simulink library "lib_plant"  (R2026a)
settings: Solver=VariableStepAuto
undefined symbols (not defined in the file or in its folder): zs0, zsdot0, zu0, zudot0
settings Model: Creator=alessandro-nardin  LastModifiedBy=alessandro-nardin

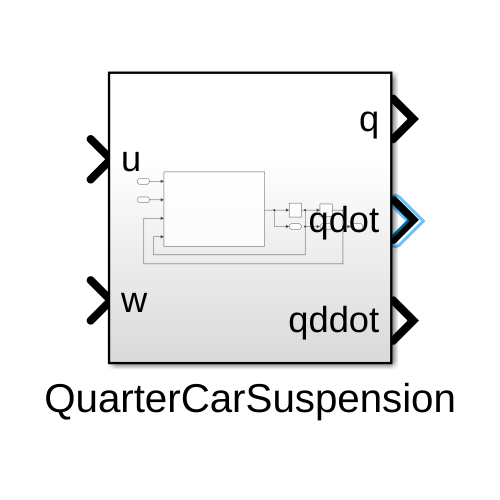
[thumbnail: Simulink's stored preview of the top-level diagram]
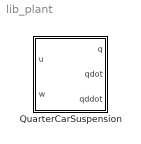
== system lib_plant ==
  QuarterCarSuspension : Subsystem

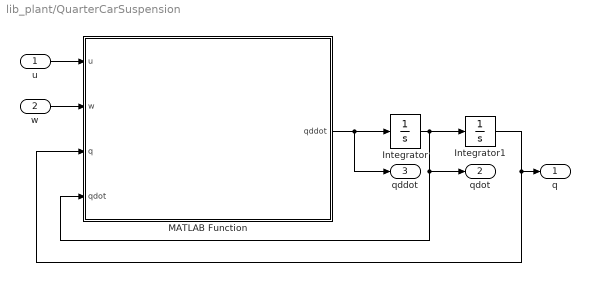
== system lib_plant/QuarterCarSuspension ==
  u : Inport
  w : Inport  Port=2
  Integrator : Integrator  InitialCondition=[ zsdot0; zudot0]
  Integrator1 : Integrator  InitialCondition=[ zs0; zu0 ]
  MATLAB Function : MATLAB Function  TreatAsAtomicUnit=on
  q : Outport
  qdot : Outport  Port=2
  qddot : Outport  Port=3
  wires:
  w/1 -> MATLAB Function/2(w)
  u/1 -> MATLAB Function/1(u)
  Integrator/1 -> qdot/1, MATLAB Function/4(qdot), Integrator1/1
  MATLAB Function/1(qddot) -> qddot/1, Integrator/1
  Integrator1/1 -> MATLAB Function/3(q), q/1

== matlab function lib_plant/QuarterCarSuspension/MATLAB Function ==
  data: u input size=[2 1]; w input size=[2 1]; q input size=[2 1]; qdot input size=[2 1]; qddot output size=[2 1]; plant_param parameter
function qddot = quarter_car_plant(u, w, q, qdot, plant_param)

    ms    = plant_param.ms;
    mu    = plant_param.mu;
    ks0   = plant_param.ks0;
    alpha = plant_param.alpha;
    bs    = plant_param.bs;
    kt    = plant_param.kt;
    bt    = plant_param.bt;

    % ESTRAZIONE INPUT
    u1 = u(1);
    u2 = u(2);

    zr    = w(1);
    zrdot = w(2);

    zs    = q(1);
    zu    = q(2);

    zsdot = qdot(1);
    zudot = qdot(2);

    % CALCOLO DELTA
    delta_s     = zs - zu;
    delta_s_dot = zsdot - zudot;
    delta_t     = zu - zr;
    delta_t_dot = zudot - zrdot;

    % CALCOLO FORZE
    Fs = ks0*delta_s + alpha*delta_s^3 + bs*delta_s_dot;
    Ft = kt*delta_t + bt*delta_t_dot;

    % SOLUZIONE
    M = [ms 0;
         0  mu];

    n = [-Fs + u1;
          Fs - Ft - u1 + u2];

    qddot = inv(M) * n;
end
